simulink library "mcm_sil_M17_52_00_03_std"  (Simulink 8.3)
settings: Solver=ode45  StartTime=0.0  StopTime=10.0  RelTol=1e-3
undefined symbols (not defined in the file): sMP
libraries: MCM21_MDEG_EURO_10ms_wrapper x1
settings Model: Creator=PBASAVA  LastModifiedBy=PBASAVA

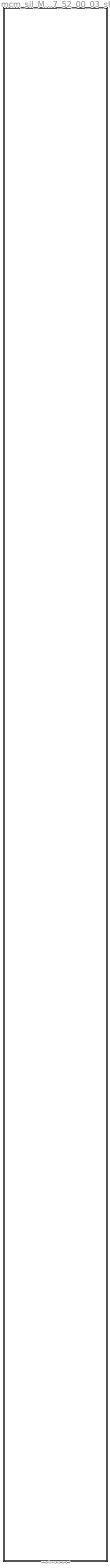
== system mcm_sil_M17_52_00_03_std ==
  mcm_sil_M17_52_00_03_std : Subsystem  mask{user_config=sMP.ctrl.mcm.user_config}

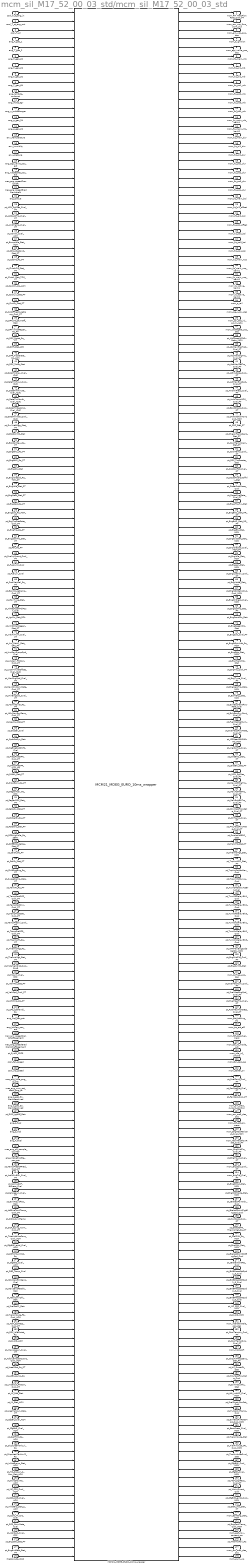
== system mcm_sil_M17_52_00_03_std/mcm_sil_M17_52_00_03_std ==
  cool_T_ct_eng_in : Inport
  cool_T_ct_eng_out : Inport  Port=2
  cool_T_oil : Inport  Port=3
  eng_T_gas_1 : Inport  Port=4
  eng_T_gas_2 : Inport  Port=5
  eng_T_gas_2N : Inport  Port=6
  eng_T_gas_2S : Inport  Port=7
  eng_T_gas_32 : Inport  Port=8
  eng_T_gas_6N : Inport  Port=9
  eng_lambda_exhaust : Inport  Port=10
  eng_mdot_egr : Inport  Port=11
  eng_n_turbocharger : Inport  Port=12
  eng_p_gas_2N : Inport  Port=13
  eng_p_gas_2S : Inport  Port=14
  env_Temperature : Inport  Port=15
  env_humidity : Inport  Port=16
  env_pressure : Inport  Port=17
  eng_egr_valve_pos_act : Inport  Port=18
  eng_wastegate_pos_act : Inport  Port=19
  mec_eng_speedCrankshaft : Inport  Port=20
  mec_eng_speedGradCrankshaft : Inport  Port=21
  eng_torque : Inport  Port=22
  pt_ACM_SglRes_Cval_PT : Inport  Port=23
  pt_ARRAddTrq_Cval_PT : Inport  Port=24
  pt_AmbTemp_Cval_PT : Inport  Port=25
  pt_AshVol_Cval_ACM : Inport  Port=26
  pt_BumpIdle_Stat_ACM : Inport  Port=27
  pt_CPC_IdleCond_Stat_PT : Inport  Port=28
  pt_CabHt_Rq_PT : Inport  Port=29
  pt_ClutchCls_Stat_PT : Inport  Port=30
  pt_Clutch_Stat_TCM_PT : Inport  Port=31
  pt_CoolDn_Rq_ACM : Inport  Port=32
  pt_CoolLvl_Stat_PT : Inport  Port=33
  pt_CurrGr_Stat_PT : Inport  Port=34
  pt_CutoffFreqSurgDamp_Cval_PT : Inport  Port=35
  pt_DPF_HC_BurnOff_Stat : Inport  Port=36
  pt_DPF_InhbtRegen_Rq_PT : Inport  Port=37
  pt_DPF_Protct_Rq_PT : Inport  Port=38
  pt_DPF_Stat_ACM : Inport  Port=39
  pt_DPF_TrqDerate_Rq_ACM : Inport  Port=40
  pt_DPF_Zone_Stat : Inport  Port=41
  pt_DateTmDay_Cval_ICUC : Inport  Port=42
  pt_DateTmHour_Cval_ICUC : Inport  Port=43
  pt_DateTmMinute_Cval_ICUC : Inport  Port=44
  pt_DateTmMonth_Cval_ICUC : Inport  Port=45
  pt_DateTmSecond_Cval_ICUC : Inport  Port=46
  pt_DateTmYear_Cval_ICUC : Inport  Port=47
  pt_DrvlineEngg_Stat_PT : Inport  Port=48
  pt_EcoRollMd_Stat : Inport  Port=49
  pt_EcoRollNeu_Rq_PT : Inport  Port=50
  pt_EngBrk1_Rq_PT : Inport  Port=51
  pt_EngBrk2_Rq_PT : Inport  Port=52
  pt_EngCrk_Stat : Inport  Port=53
  pt_EngIdleSpd_Rq_TCM_PT : Inport  Port=54
  pt_EngIdle_Stat_PT : Inport  Port=55
  pt_EngReSt_Stat_PT : Inport  Port=56
  pt_EngSpd_Rq_PT : Inport  Port=57
  pt_EngSpd_Rq_TCM_PT : Inport  Port=58
  pt_EngTrqDecRate_Cval_PT : Inport  Port=59
  pt_EngTrq_Rq_PT : Inport  Port=60
  pt_EngZeroTrq_Stat_PT : Inport  Port=61
  pt_Fan_Rq_PT : Inport  Port=62
  pt_FuelInjQuant_Cval_PT : Inport  Port=63
  pt_FuelLvl2_Cval : Inport  Port=64
  pt_FuelLvl_Cval : Inport  Port=65
  pt_FuelMapSel_Rq_PT : Inport  Port=66
  pt_GaimSurgDamp_Cval_PT : Inport  Port=67
  pt_GovType_Stat_PT : Inport  Port=68
  pt_HiResAccelPdlPosn_Cval : Inport  Port=69
  pt_IgnSw_Stat_SCA : Inport  Port=70
  pt_InhbtManRegen_Stat_PT : Inport  Port=71
  pt_IntkAirHum_Cval_PT : Inport  Port=72
  pt_Km_Parity_Stat_CPC_PT : Inport  Port=73
  pt_LimGovDroopSpd_Cval : Inport  Port=74
  pt_LmdaIn_FltrCorr_Cval_PT : Inport  Port=75
  pt_LocalMinuteOffset_Cval_ICUC : Inport  Port=76
  pt_MaxEngSpd_Cval_PT : Inport  Port=77
  pt_MaxNOxConvRate_Cval_PT : Inport  Port=78
  pt_MinEngSpd_Cval_PT : Inport  Port=79
  pt_MomntOver_Rq_PT : Inport  Port=80
  pt_NOxRawEmiSens_Cval_PT : Inport  Port=81
  pt_NeuSw_Stat_PT : Inport  Port=82
  pt_ObsSel_Cval : Inport  Port=83
  pt_OptIdleSys_Stat : Inport  Port=84
  pt_PreEngSpdShift_Cval : Inport  Port=85
  pt_PressPostDPF_Cval_PT : Inport  Port=86
  pt_PressPreDPF_Cval_PT : Inport  Port=87
  pt_PrkBrk_Stat_PT : Inport  Port=88
  pt_PropGain_Rq_PT : Inport  Port=89
  pt_RegenActv_Rq_CPC : Inport  Port=90
  pt_RegenDPF_Stat_PT : Inport  Port=91
  pt_RetActv_Stat_PT : Inport  Port=92
  pt_RlsSelGr_Rq_PT : Inport  Port=93
  pt_RotSens_Stat_PT : Inport  Port=94
  pt_SCRHighIdle_Rq_SERV : Inport  Port=95
  pt_SPEEDO_ZeSig_Stat_PT : Inport  Port=96
  pt_SelGr_Rq_PT : Inport  Port=97
  pt_SelGr_Stat_PT : Inport  Port=98
  pt_ShiftSprtEng_Rq_PT : Inport  Port=99
  pt_SurgeDamp_Stat_PT : Inport  Port=100
  pt_TankHt_Rq_PT : Inport  Port=101
  pt_TempPostDPF_Cval_PT : Inport  Port=102
  pt_TempPostOxi_Cval_PT : Inport  Port=103
  pt_TempPostSCR_Cval_PT : Inport  Port=104
  pt_TempPreOxi_Cval_PT : Inport  Port=105
  pt_TempPreSCR_Cval_PT : Inport  Port=106
  pt_ThermoHt_Rq_PT : Inport  Port=107
  pt_ThermoMgt_Rq_ACM : Inport  Port=108
  pt_ThermoMgt_Stat_PT : Inport  Port=109
  pt_TotalVehDist_Cval_DIAG : Inport  Port=110
  pt_TrqLim_Cval_CPC : Inport  Port=111
  pt_VehMtn_Stat_PT : Inport  Port=112
  pt_VehSpd_Cval_PT : Inport  Port=113
  pt_WtrPmp_Rq_PT : Inport  Port=114
  pt_ZPC_CstHandl_Rq : Inport  Port=115
  eng_vcp_pos_act : Inport  Port=116
  eng_brkflap_pos_act : Inport  Port=117
  mec_eng_speedCrankshaftSegment : Inport  Port=118
  mec_eng_speedGradCrankshaftSegment : Inport  Port=119
  pt_SysID_CPC3 : Inport  Port=120
  cool_fan_speed : Inport  Port=121
  cool_wp_speed : Inport  Port=122
  mec_eng_time_ang_cs_act : Inport  Port=123
  mec_eng_num_act_tooth_ang_cs : Inport  Port=124
  eng_p_gas_31_CrankResolved : Inport  Port=125
  eng_p_gas_32_CrankResolved : Inport  Port=126
  pt_DOC_LgtOff_Stat : Inport  Port=127
  eng_p_fuel : Inport  Port=128
  eng_p_hcd : Inport  Port=129
  eng_T_Fuel : Inport  Port=130
  mec_eng_p3_sample_counter : Inport  Port=131
  eng_intakethrottle_pos_act : Inport  Port=132
  pt_TempPreSCRPred_Cval_PT : Inport  Port=133
  pt_ActlNOxEmi_Cval_PT : Inport  Port=134
  pt_Norm_DPF_BkPress_Cval : Inport  Port=135
  pt_RelUreaLvl_Cval_PT : Inport  Port=136
  pt_ExhHtSysFlap_Stat : Inport  Port=137
  pt_AdBlueTankTemp_Cval_PT : Inport  Port=138
  pt_DOC_SyncTemp : Inport  Port=139
  pt_SCR_aging_norm_Cval_PT : Inport  Port=140
  pt_TotalAdblueCons_Cval_ACM : Inport  Port=141
  pt_CfgBit2_extd_Cval_ACM : Inport  Port=142
  pt_DPF_HC_Inhbt_Rq : Inport  Port=143
  pt_CfgBit2_Cval_ACM : Inport  Port=144
  pt_DEF_Temp_Cval : Inport  Port=145
  pt_NOxRawEmiSens_Cval : Inport  Port=146
  pt_NOxSensRatChk_Stat : Inport  Port=147
  pt_NOxConvChk_Stat : Inport  Port=148
  pt_FuelRefill_Stat : Inport  Port=149
  pt_Tier4Induce_FR_Cval_ACM : Inport  Port=150
  pt_ACM_SglRes2_Cval_PT : Inport  Port=151
  pt_DPF_IdleProtct_Rq : Inport  Port=152
  pt_SysID_ACM : Inport  Port=153
  pt_MaxUreaLvl_Cval_PT : Inport  Port=154
  pt_AdblueDoserQuant_Cval_ACM : Inport  Port=155
  pt_UreaDfrst_Rq_PT : Inport  Port=156
  pt_AdBlueLmp_Rq : Inport  Port=157
  pt_LmdaOut_FltrCorr_Cval_PT : Inport  Port=158
  pt_MI_Rds_Stat : Inport  Port=159
  pt_MI_Stat_ACM : Inport  Port=160
  pt_UreaTankLvl_Stat_PT : Inport  Port=161
  pt_CfgBit_Cval_ACM : Inport  Port=162
  pt_CfgBit3_Cval_ACM : Inport  Port=163
  pt_DelFMM_Rq_ACM : Inport  Port=164
  pt_DispUreaTankLvl_Rq : Inport  Port=165
  pt_DispUreaTankLvl2_Rq : Inport  Port=166
  pt_InhbtGroup_Stat_ACM : Inport  Port=167
  pt_HC_DosLvl_2_Mon_Stat_ACM : Inport  Port=168
  pt_FuncSftyVer_ACM : Inport  Port=169
  pt_MC_C29_Cval_ACM : Inport  Port=170
  pt_CRC_C29_Cval_ACM : Inport  Port=171
  pt_InhbtGrp_Stat_2_ACM : Inport  Port=172
  pt_Cont_MI_Cnt_Cval : Inport  Port=173
  pt_SCR_ConvRate_Cval : Inport  Port=174
  pt_VehSpd_Cval_CPC : Inport  Port=175
  pt_EngStrtr_Stat_PT : Inport  Port=176
  pt_EngExtStart_Stat_PT : Inport  Port=177
  PressAir_Rq_ICUC : Inport  Port=178
  MCM21_MDEG_EURO_10ms_wrapper : MCM21_MDEG_EURO_10ms_wrapper/MCM21_MDEG_EURO_10ms_wrapper  SystemSampleTime=-1
  mcm_PM_MassFlowRate_Cval_PT : Outport
  mcm_am_vcp_5ms_pwm_out : Outport  Port=2
  mcm_am_vcp_pos_des : Outport  Port=3
  mcm_b_ignition : Outport  Port=4
  mcm_egr_valve_pos_des : Outport  Port=5
  mcm_fis_main_mb : Outport  Port=6
  mcm_fis_pi1_mb : Outport  Port=7
  mcm_fis_pi2_mb : Outport  Port=8
  mcm_fis_po1_mb : Outport  Port=9
  mcm_fis_po2_mb : Outport  Port=10
  mcm_fis_po3_mb : Outport  Port=11
  mcm_fis_po4_mb : Outport  Port=12
  mcm_fis_main_mb_bank1 : Outport  Port=13
  mcm_fis_main_mb_bank2 : Outport  Port=14
  mcm_fis_main_dur : Outport  Port=15
  mcm_fis_pi1_dur : Outport  Port=16
  mcm_fis_pi2_dur : Outport  Port=17
  mcm_fis_po1_dur : Outport  Port=18
  mcm_fis_po2_dur : Outport  Port=19
  mcm_fis_po3_dur : Outport  Port=20
  mcm_fis_po4_dur : Outport  Port=21
  mcm_fis_main_boi : Outport  Port=22
  mcm_fis_pi1_offset : Outport  Port=23
  mcm_fis_pi2_boi : Outport  Port=24
  mcm_fis_po1_offset : Outport  Port=25
  mcm_fis_po2_boi : Outport  Port=26
  mcm_fis_po3_boi : Outport  Port=27
  mcm_fis_po4_boi : Outport  Port=28
  mcm_fis_main_nop : Outport  Port=29
  mcm_fis_main_nop_bank1 : Outport  Port=30
  mcm_fis_main_nop_bank2 : Outport  Port=31
  mcm_jb_active_bank1 : Outport  Port=32
  mcm_jb_active_bank2 : Outport  Port=33
  mcm_p_rail : Outport  Port=34
  mcm_rpg_i_pcv_des : Outport  Port=35
  mcm_spi_des_inj_asym_ratio : Outport  Port=36
  mcm_wastegate_pos_des : Outport  Port=37
  pt_ANCReadWFNOxRatio_MCM : Outport  Port=38
  pt_AbsMaxEngTrq2_Cval_PT : Outport  Port=39
  pt_AbsMaxEngTrq_Cval_PT : Outport  Port=40
  pt_AbsMaxRetTrq_Cval_PT : Outport  Port=41
  pt_ActlInjRate_Cval_PT : Outport  Port=42
  pt_ActlMaxEngSpd_Cval_PT : Outport  Port=43
  pt_AmbAirPress_Cval_PT : Outport  Port=44
  pt_AmbTempMCM_Cval_PT : Outport  Port=45
  pt_BoostPress_Cval_PT : Outport  Port=46
  pt_CANWrtGlblMonCond_MCM : Outport  Port=47
  pt_CPC_Stat_PT : Outport  Port=48
  pt_ChrgAirTempSens_Stat_PT : Outport  Port=49
  pt_CoolTempWarn_Stat_PT : Outport  Port=50
  pt_CoolTemp_Cval_PT : Outport  Port=51
  pt_DPF_TrqDerate_Stat : Outport  Port=52
  pt_DosCorrFctr_Cval_PT : Outport  Port=53
  pt_DoserFuelCutoffVlv_Stat : Outport  Port=54
  pt_DoserFuelPress_Cval : Outport  Port=55
  pt_DoserFuelRate_Cval_PT : Outport  Port=56
  pt_EngATS_Hw_Stat : Outport  Port=57
  pt_EngBrk1_Stat_MR_PT : Outport  Port=58
  pt_EngBrk2_Stat_MR_PT : Outport  Port=59
  pt_EngBrk_Stat_MCM : Outport  Port=60
  pt_EngExtStart_Stat_MCM : Outport  Port=61
  pt_EngIdleSpd_Cval_MCM_PT : Outport  Port=62
  pt_EngIdle_Stat_MCM : Outport  Port=63
  pt_EngIgn_Stat_MCM : Outport  Port=64
  pt_EngLoadIdx_Cval_PT : Outport  Port=65
  pt_EngMode_Stat_MCM : Outport  Port=66
  pt_EngNO2RatioOut_Cval_MCM : Outport  Port=67
  pt_EngOilPress_Cval_MCM : Outport  Port=68
  pt_EngOpPnt_Stat_PT : Outport  Port=69
  pt_EngPendRls_Stat : Outport  Port=70
  pt_EngRegenRls_Stat : Outport  Port=71
  pt_EngSpd_Cval_PT : Outport  Port=72
  pt_EngStSpInhbt_Rq_MCM : Outport  Port=73
  pt_EngStrtr_Stat_MCM : Outport  Port=74
  pt_EngTransMd_Stat : Outport  Port=75
  pt_EngTrq_Cval_PT : Outport  Port=76
  pt_EngType_Cval_PT : Outport  Port=77
  pt_EngZeroTrq_Stat_MCM : Outport  Port=78
  pt_EomEng_Stat_MCM : Outport  Port=79
  pt_ExhGasMassFlowRate_Cval : Outport  Port=80
  pt_ExhGasOxyCont_Cval_PT : Outport  Port=81
  pt_FuelMapSelNum_Cval_PT : Outport  Port=82
  pt_FuelMassFlowRate_Cval_PT : Outport  Port=83
  pt_ISPRead30GNOxMd_MCM : Outport  Port=84
  pt_InertiaTrq_Cval_PT : Outport  Port=85
  pt_JakeBrk2_Stat_PT : Outport  Port=86
  pt_JakeBrk_Stat_PT : Outport  Port=87
  pt_MCM_SglRes_Cval_PT : Outport  Port=88
  pt_MaxActlEngTrq_Cval_PT : Outport  Port=89
  pt_MaxActlRetTrq_Cval_PT : Outport  Port=90
  pt_MaxEngBrkTrq_Cval_PT : Outport  Port=91
  pt_NOxMassFlowRate_Cval_PT : Outport  Port=92
  pt_OilTemp_Cval_PT : Outport  Port=93
  pt_PM_MassFlowRate_Cval_PT : Outport  Port=94
  pt_SmokeMdEOP_Stat : Outport  Port=95
  pt_TankHt_Stat_PT : Outport  Port=96
  pt_ThermoMgt_Stat_MCM : Outport  Port=97
  pt_TrqLimNOx_Stat_PT : Outport  Port=98
  pt_TrqLimPctAbsMax_Cval : Outport  Port=99
  pt_TrqLimPctCurve_Cval : Outport  Port=100
  pt_TurnOffDelayActBrk_Cval : Outport  Port=101
  pt_TurnOffDelayBrk1_Cval : Outport  Port=102
  pt_TurnOffDelayBrk2_Cval : Outport  Port=103
  pt_TurnOffDelayBrk3_Cval : Outport  Port=104
  pt_TurnOnDelayBrk1_Cval : Outport  Port=105
  pt_TurnOnDelayBrk2_Cval : Outport  Port=106
  pt_TurnOnDelayBrk3_Cval : Outport  Port=107
  pt_WFAMaxEngSpd30gNOx_MCM : Outport  Port=108
  pt_EngFrictTrq_Cval_PT : Outport  Port=109
  pt_EngCylMd_Stat : Outport  Port=110
  mcm_brkflap_pos_des : Outport  Port=111
  pt_FuelMapNum_Cval_PT : Outport  Port=112
  pt_FuelMapEngSpd_Cval_PT : Outport  Port=113
  pt_FuelMapTrq_Cval_PT : Outport  Port=114
  pt_FuelMapTrqNoBst_Cval_PT : Outport  Port=115
  mcm_act_braking_trq : Outport  Port=116
  mcm_trq_act_eff : Outport  Port=117
  mcm_fbf_des_fuel_mass : Outport  Port=118
  mcm_tsa_itc_mode_act : Outport  Port=119
  mcm_wfa_wf_smoke : Outport  Port=120
  mcm_fan_spd_req : Outport  Port=121
  mcm_starter_on : Outport  Port=122
  pt_FuelCons_Cval_PT : Outport  Port=123
  pt_FanSpdPct_Cval_PT : Outport  Port=124
  pt_FanSpd_Cval_PT : Outport  Port=125
  mcm_am_sra3_current_position : Outport  Port=126
  mcm_am_sra3_des_pos : Outport  Port=127
  mcm_ccf_act_air_mass : Outport  Port=128
  mcm_EngNO2RatioOut_Cval_MCM : Outport  Port=129
  mcm_NOxMassFlowRate_Cval_PT : Outport  Port=130
  mcm_EngFrictTrq_Cval_PT : Outport  Port=131
  pt_EngHours_Cval_PT : Outport  Port=132
  mcm_EngSpd_Cval_PT : Outport  Port=133
  mcm_EngTrq_Cval_PT : Outport  Port=134
  pt_EngStrtrLk_Stat_MCM : Outport  Port=135
  pt_EngStrtrMode_Stat_MCM : Outport  Port=136
  pt_JBrakeSPointIdx_Cval : Outport  Port=137
  pt_JBrakeSPointTrgtEngSpd_Cval : Outport  Port=138
  pt_PwrClass_Cval_PT : Outport  Port=139
  pt_DeactDPF_ThermoMgt_Rq_PT : Outport  Port=140
  pt_DelFMM_Rq_MCM : Outport  Port=141
  pt_EngSNA_Stat_MCM : Outport  Port=142
  pt_JBrakeSPointStrtEngSpd_Cval : Outport  Port=143
  pt_JBrakeWghtFac_Cval : Outport  Port=144
  pt_JBrkBPressStrtSpd1_3_Cval : Outport  Port=145
  pt_JBrkBPressStrtSpd1_6_Cval : Outport  Port=146
  pt_JBrkBPressStrtSpd2_3_Cval : Outport  Port=147
  pt_JBrkBPressStrtSpd2_6_Cval : Outport  Port=148
  pt_MC_C02_Cval_MCM : Outport  Port=149
  pt_SysID_MCM : Outport  Port=150
  mcm_intakethrottle_pos_des : Outport  Port=151
  pt_CoolTempIn_Cval_PT : Outport  Port=152
  pt_CoolTempOut_Cval_PT : Outport  Port=153
  mcm_mdot_SFI : Outport  Port=154
  pt_ChrgAirPressSens_Stat_PT : Outport  Port=155
  pt_HC_DoserFlt_Stat : Outport  Port=156
  pt_PM_MassFlowRate_Cval : Outport  Port=157
  pt_ExhHtSysRls_Stat : Outport  Port=158
  pt_At1_IntkO2_Cval_MCM : Outport  Port=159
  pt_FuelDnstyCorrFctr_Cval : Outport  Port=160
  pt_TurboOutTemp_Cval : Outport  Port=161
  pt_ExhGasFlwRateMod_Cval_MCM : Outport  Port=162
  pt_BaroPress_Cval_MCM : Outport  Port=163
  pt_Tier4Induce_Stat : Outport  Port=164
  pt_Tier4Induce_FR_Cval_MCM : Outport  Port=165
  pt_Tier4InduceOvrd_Stat : Outport  Port=166
  pt_CfgBit2_Cval_MCM : Outport  Port=167
  pt_CfgBit_Cval_MCM : Outport  Port=168
  pt_MCM_SglRes2_Cval_PT : Outport  Port=169
  pt_WtrInjQuant_Cval : Outport  Port=170
  pt_CfgBit2_extd_Cval_MCM : Outport  Port=171
  pt_DEF_Lmp_Stat_PT : Outport  Port=172
  mcm_EomEng_Stat_MCM : Outport  Port=173
  pt_EngCoolTemp_Cval_MCM : Outport  Port=174
  mcm_eaf_nox_content_cor : Outport  Port=175
  pt_ThermoRoll_Rq : Outport  Port=176
  mcm_am_sra4_des_pos : Outport  Port=177
  mcm_pwm_wp : Outport  Port=178
  wires:
  cool_T_ct_eng_in/1 -> MCM21_MDEG_EURO_10ms_wrapper/1  "cool_T_ct_eng_in"
  cool_T_ct_eng_out/1 -> MCM21_MDEG_EURO_10ms_wrapper/2  "cool_T_ct_eng_out"
  cool_T_oil/1 -> MCM21_MDEG_EURO_10ms_wrapper/3  "cool_T_oil"
  eng_T_gas_1/1 -> MCM21_MDEG_EURO_10ms_wrapper/4  "eng_T_gas_1"
  eng_T_gas_2/1 -> MCM21_MDEG_EURO_10ms_wrapper/5  "eng_T_gas_2"
  eng_T_gas_2N/1 -> MCM21_MDEG_EURO_10ms_wrapper/6  "eng_T_gas_2N"
  eng_T_gas_2S/1 -> MCM21_MDEG_EURO_10ms_wrapper/7  "eng_T_gas_2S"
  eng_T_gas_32/1 -> MCM21_MDEG_EURO_10ms_wrapper/8  "eng_T_gas_32"
  eng_T_gas_6N/1 -> MCM21_MDEG_EURO_10ms_wrapper/9  "eng_T_gas_6N"
  eng_lambda_exhaust/1 -> MCM21_MDEG_EURO_10ms_wrapper/10  "eng_lambda_exhaust"
  eng_mdot_egr/1 -> MCM21_MDEG_EURO_10ms_wrapper/11  "eng_mdot_egr"
  eng_n_turbocharger/1 -> MCM21_MDEG_EURO_10ms_wrapper/12  "eng_n_turbocharger"
  eng_p_gas_2N/1 -> MCM21_MDEG_EURO_10ms_wrapper/13  "eng_p_gas_2N"
  eng_p_gas_2S/1 -> MCM21_MDEG_EURO_10ms_wrapper/14  "eng_p_gas_2S"
  env_Temperature/1 -> MCM21_MDEG_EURO_10ms_wrapper/15  "env_Temperature"
  env_humidity/1 -> MCM21_MDEG_EURO_10ms_wrapper/16  "env_humidity"
  env_pressure/1 -> MCM21_MDEG_EURO_10ms_wrapper/17  "env_pressure"
  eng_egr_valve_pos_act/1 -> MCM21_MDEG_EURO_10ms_wrapper/18  "eng_egr_valve_pos_act"
  eng_wastegate_pos_act/1 -> MCM21_MDEG_EURO_10ms_wrapper/19  "eng_wastegate_pos_act"
  mec_eng_speedCrankshaft/1 -> MCM21_MDEG_EURO_10ms_wrapper/20  "mec_eng_speedCrankshaft"
  mec_eng_speedGradCrankshaft/1 -> MCM21_MDEG_EURO_10ms_wrapper/21  "mec_eng_speedGradCrankshaft"
  eng_torque/1 -> MCM21_MDEG_EURO_10ms_wrapper/22  "eng_torque"
  pt_ACM_SglRes_Cval_PT/1 -> MCM21_MDEG_EURO_10ms_wrapper/23  "pt_ACM_SglRes_Cval_PT"
  pt_ARRAddTrq_Cval_PT/1 -> MCM21_MDEG_EURO_10ms_wrapper/24  "pt_ARRAddTrq_Cval_PT"
  pt_AmbTemp_Cval_PT/1 -> MCM21_MDEG_EURO_10ms_wrapper/25  "pt_AmbTemp_Cval_PT"
  pt_AshVol_Cval_ACM/1 -> MCM21_MDEG_EURO_10ms_wrapper/26  "pt_AshVol_Cval_ACM"
  pt_BumpIdle_Stat_ACM/1 -> MCM21_MDEG_EURO_10ms_wrapper/27  "pt_BumpIdle_Stat_ACM"
  pt_CPC_IdleCond_Stat_PT/1 -> MCM21_MDEG_EURO_10ms_wrapper/28  "pt_CPC_IdleCond_Stat_PT"
  pt_CabHt_Rq_PT/1 -> MCM21_MDEG_EURO_10ms_wrapper/29  "pt_CabHt_Rq_PT"
  pt_ClutchCls_Stat_PT/1 -> MCM21_MDEG_EURO_10ms_wrapper/30  "pt_ClutchCls_Stat_PT"
  pt_Clutch_Stat_TCM_PT/1 -> MCM21_MDEG_EURO_10ms_wrapper/31  "pt_Clutch_Stat_TCM_PT"
  pt_CoolDn_Rq_ACM/1 -> MCM21_MDEG_EURO_10ms_wrapper/32  "pt_CoolDn_Rq_ACM"
  pt_CoolLvl_Stat_PT/1 -> MCM21_MDEG_EURO_10ms_wrapper/33  "pt_CoolLvl_Stat_PT"
  pt_CurrGr_Stat_PT/1 -> MCM21_MDEG_EURO_10ms_wrapper/34  "pt_CurrGr_Stat_PT"
  pt_CutoffFreqSurgDamp_Cval_PT/1 -> MCM21_MDEG_EURO_10ms_wrapper/35  "pt_CutoffFreqSurgDamp_Cval_PT"
  pt_DPF_HC_BurnOff_Stat/1 -> MCM21_MDEG_EURO_10ms_wrapper/36  "pt_DPF_HC_BurnOff_Stat"
  pt_DPF_InhbtRegen_Rq_PT/1 -> MCM21_MDEG_EURO_10ms_wrapper/37  "pt_DPF_InhbtRegen_Rq_PT"
  pt_DPF_Protct_Rq_PT/1 -> MCM21_MDEG_EURO_10ms_wrapper/38  "pt_DPF_Protct_Rq_PT"
  pt_DPF_Stat_ACM/1 -> MCM21_MDEG_EURO_10ms_wrapper/39  "pt_DPF_Stat_ACM"
  pt_DPF_TrqDerate_Rq_ACM/1 -> MCM21_MDEG_EURO_10ms_wrapper/40  "pt_DPF_TrqDerate_Rq_ACM"
  pt_DPF_Zone_Stat/1 -> MCM21_MDEG_EURO_10ms_wrapper/41  "pt_DPF_Zone_Stat"
  pt_DateTmDay_Cval_ICUC/1 -> MCM21_MDEG_EURO_10ms_wrapper/42  "pt_DateTmDay_Cval_ICUC"
  pt_DateTmHour_Cval_ICUC/1 -> MCM21_MDEG_EURO_10ms_wrapper/43  "pt_DateTmHour_Cval_ICUC"
  pt_DateTmMinute_Cval_ICUC/1 -> MCM21_MDEG_EURO_10ms_wrapper/44  "pt_DateTmMinute_Cval_ICUC"
  pt_DateTmMonth_Cval_ICUC/1 -> MCM21_MDEG_EURO_10ms_wrapper/45  "pt_DateTmMonth_Cval_ICUC"
  pt_DateTmSecond_Cval_ICUC/1 -> MCM21_MDEG_EURO_10ms_wrapper/46  "pt_DateTmSecond_Cval_ICUC"
  pt_DateTmYear_Cval_ICUC/1 -> MCM21_MDEG_EURO_10ms_wrapper/47  "pt_DateTmYear_Cval_ICUC"
  pt_DrvlineEngg_Stat_PT/1 -> MCM21_MDEG_EURO_10ms_wrapper/48  "pt_DrvlineEngg_Stat_PT"
  pt_EcoRollMd_Stat/1 -> MCM21_MDEG_EURO_10ms_wrapper/49  "pt_EcoRollMd_Stat"
  pt_EcoRollNeu_Rq_PT/1 -> MCM21_MDEG_EURO_10ms_wrapper/50  "pt_EcoRollNeu_Rq_PT"
  pt_EngBrk1_Rq_PT/1 -> MCM21_MDEG_EURO_10ms_wrapper/51  "pt_EngBrk1_Rq_PT"
  pt_EngBrk2_Rq_PT/1 -> MCM21_MDEG_EURO_10ms_wrapper/52  "pt_EngBrk2_Rq_PT"
  pt_EngCrk_Stat/1 -> MCM21_MDEG_EURO_10ms_wrapper/53  "pt_EngCrk_Stat"
  pt_EngIdleSpd_Rq_TCM_PT/1 -> MCM21_MDEG_EURO_10ms_wrapper/54  "pt_EngIdleSpd_Rq_TCM_PT"
  pt_EngIdle_Stat_PT/1 -> MCM21_MDEG_EURO_10ms_wrapper/55  "pt_EngIdle_Stat_PT"
  pt_EngReSt_Stat_PT/1 -> MCM21_MDEG_EURO_10ms_wrapper/56  "pt_EngReSt_Stat_PT"
  pt_EngSpd_Rq_PT/1 -> MCM21_MDEG_EURO_10ms_wrapper/57  "pt_EngSpd_Rq_PT"
  pt_EngSpd_Rq_TCM_PT/1 -> MCM21_MDEG_EURO_10ms_wrapper/58  "pt_EngSpd_Rq_TCM_PT"
  pt_EngTrqDecRate_Cval_PT/1 -> MCM21_MDEG_EURO_10ms_wrapper/59  "pt_EngTrqDecRate_Cval_PT"
  pt_EngTrq_Rq_PT/1 -> MCM21_MDEG_EURO_10ms_wrapper/60  "pt_EngTrq_Rq_PT"
  pt_EngZeroTrq_Stat_PT/1 -> MCM21_MDEG_EURO_10ms_wrapper/61  "pt_EngZeroTrq_Stat_PT"
  pt_Fan_Rq_PT/1 -> MCM21_MDEG_EURO_10ms_wrapper/62  "pt_Fan_Rq_PT"
  pt_FuelInjQuant_Cval_PT/1 -> MCM21_MDEG_EURO_10ms_wrapper/63  "pt_FuelInjQuant_Cval_PT"
  pt_FuelLvl2_Cval/1 -> MCM21_MDEG_EURO_10ms_wrapper/64  "pt_FuelLvl2_Cval"
  pt_FuelLvl_Cval/1 -> MCM21_MDEG_EURO_10ms_wrapper/65  "pt_FuelLvl_Cval"
  pt_FuelMapSel_Rq_PT/1 -> MCM21_MDEG_EURO_10ms_wrapper/66  "pt_FuelMapSel_Rq_PT"
  pt_GaimSurgDamp_Cval_PT/1 -> MCM21_MDEG_EURO_10ms_wrapper/67  "pt_GaimSurgDamp_Cval_PT"
  pt_GovType_Stat_PT/1 -> MCM21_MDEG_EURO_10ms_wrapper/68  "pt_GovType_Stat_PT"
  pt_HiResAccelPdlPosn_Cval/1 -> MCM21_MDEG_EURO_10ms_wrapper/69  "pt_HiResAccelPdlPosn_Cval"
  pt_IgnSw_Stat_SCA/1 -> MCM21_MDEG_EURO_10ms_wrapper/70  "pt_IgnSw_Stat_SCA"
  pt_InhbtManRegen_Stat_PT/1 -> MCM21_MDEG_EURO_10ms_wrapper/71  "pt_InhbtManRegen_Stat_PT"
  pt_IntkAirHum_Cval_PT/1 -> MCM21_MDEG_EURO_10ms_wrapper/72  "pt_IntkAirHum_Cval_PT"
  pt_Km_Parity_Stat_CPC_PT/1 -> MCM21_MDEG_EURO_10ms_wrapper/73  "pt_Km_Parity_Stat_CPC_PT"
  pt_LimGovDroopSpd_Cval/1 -> MCM21_MDEG_EURO_10ms_wrapper/74  "pt_LimGovDroopSpd_Cval"
  pt_LmdaIn_FltrCorr_Cval_PT/1 -> MCM21_MDEG_EURO_10ms_wrapper/75  "pt_LmdaIn_FltrCorr_Cval_PT"
  pt_LocalMinuteOffset_Cval_ICUC/1 -> MCM21_MDEG_EURO_10ms_wrapper/76  "pt_LocalMinuteOffset_Cval_ICUC"
  pt_MaxEngSpd_Cval_PT/1 -> MCM21_MDEG_EURO_10ms_wrapper/77  "pt_MaxEngSpd_Cval_PT"
  pt_MaxNOxConvRate_Cval_PT/1 -> MCM21_MDEG_EURO_10ms_wrapper/78  "pt_MaxNOxConvRate_Cval_PT"
  pt_MinEngSpd_Cval_PT/1 -> MCM21_MDEG_EURO_10ms_wrapper/79  "pt_MinEngSpd_Cval_PT"
  pt_MomntOver_Rq_PT/1 -> MCM21_MDEG_EURO_10ms_wrapper/80  "pt_MomntOver_Rq_PT"
  pt_NOxRawEmiSens_Cval_PT/1 -> MCM21_MDEG_EURO_10ms_wrapper/81  "pt_NOxRawEmiSens_Cval_PT"
  pt_NeuSw_Stat_PT/1 -> MCM21_MDEG_EURO_10ms_wrapper/82  "pt_NeuSw_Stat_PT"
  pt_ObsSel_Cval/1 -> MCM21_MDEG_EURO_10ms_wrapper/83  "pt_ObsSel_Cval"
  pt_OptIdleSys_Stat/1 -> MCM21_MDEG_EURO_10ms_wrapper/84  "pt_OptIdleSys_Stat"
  pt_PreEngSpdShift_Cval/1 -> MCM21_MDEG_EURO_10ms_wrapper/85  "pt_PreEngSpdShift_Cval"
  pt_PressPostDPF_Cval_PT/1 -> MCM21_MDEG_EURO_10ms_wrapper/86  "pt_PressPostDPF_Cval_PT"
  pt_PressPreDPF_Cval_PT/1 -> MCM21_MDEG_EURO_10ms_wrapper/87  "pt_PressPreDPF_Cval_PT"
  pt_PrkBrk_Stat_PT/1 -> MCM21_MDEG_EURO_10ms_wrapper/88  "pt_PrkBrk_Stat_PT"
  pt_PropGain_Rq_PT/1 -> MCM21_MDEG_EURO_10ms_wrapper/89  "pt_PropGain_Rq_PT"
  pt_RegenActv_Rq_CPC/1 -> MCM21_MDEG_EURO_10ms_wrapper/90  "pt_RegenActv_Rq_CPC"
  pt_RegenDPF_Stat_PT/1 -> MCM21_MDEG_EURO_10ms_wrapper/91  "pt_RegenDPF_Stat_PT"
  pt_RetActv_Stat_PT/1 -> MCM21_MDEG_EURO_10ms_wrapper/92  "pt_RetActv_Stat_PT"
  pt_RlsSelGr_Rq_PT/1 -> MCM21_MDEG_EURO_10ms_wrapper/93  "pt_RlsSelGr_Rq_PT"
  pt_RotSens_Stat_PT/1 -> MCM21_MDEG_EURO_10ms_wrapper/94  "pt_RotSens_Stat_PT"
  pt_SCRHighIdle_Rq_SERV/1 -> MCM21_MDEG_EURO_10ms_wrapper/95  "pt_SCRHighIdle_Rq_SERV"
  pt_SPEEDO_ZeSig_Stat_PT/1 -> MCM21_MDEG_EURO_10ms_wrapper/96  "pt_SPEEDO_ZeSig_Stat_PT"
  pt_SelGr_Rq_PT/1 -> MCM21_MDEG_EURO_10ms_wrapper/97  "pt_SelGr_Rq_PT"
  pt_SelGr_Stat_PT/1 -> MCM21_MDEG_EURO_10ms_wrapper/98  "pt_SelGr_Stat_PT"
  pt_ShiftSprtEng_Rq_PT/1 -> MCM21_MDEG_EURO_10ms_wrapper/99  "pt_ShiftSprtEng_Rq_PT"
  pt_SurgeDamp_Stat_PT/1 -> MCM21_MDEG_EURO_10ms_wrapper/100  "pt_SurgeDamp_Stat_PT"
  pt_TankHt_Rq_PT/1 -> MCM21_MDEG_EURO_10ms_wrapper/101  "pt_TankHt_Rq_PT"
  pt_TempPostDPF_Cval_PT/1 -> MCM21_MDEG_EURO_10ms_wrapper/102  "pt_TempPostDPF_Cval_PT"
  pt_TempPostOxi_Cval_PT/1 -> MCM21_MDEG_EURO_10ms_wrapper/103  "pt_TempPostOxi_Cval_PT"
  pt_TempPostSCR_Cval_PT/1 -> MCM21_MDEG_EURO_10ms_wrapper/104  "pt_TempPostSCR_Cval_PT"
  pt_TempPreOxi_Cval_PT/1 -> MCM21_MDEG_EURO_10ms_wrapper/105  "pt_TempPreOxi_Cval_PT"
  pt_TempPreSCR_Cval_PT/1 -> MCM21_MDEG_EURO_10ms_wrapper/106  "pt_TempPreSCR_Cval_PT"
  pt_ThermoHt_Rq_PT/1 -> MCM21_MDEG_EURO_10ms_wrapper/107  "pt_ThermoHt_Rq_PT"
  pt_ThermoMgt_Rq_ACM/1 -> MCM21_MDEG_EURO_10ms_wrapper/108  "pt_ThermoMgt_Rq_ACM"
  pt_ThermoMgt_Stat_PT/1 -> MCM21_MDEG_EURO_10ms_wrapper/109  "pt_ThermoMgt_Stat_PT"
  pt_TotalVehDist_Cval_DIAG/1 -> MCM21_MDEG_EURO_10ms_wrapper/110  "pt_TotalVehDist_Cval_DIAG"
  pt_TrqLim_Cval_CPC/1 -> MCM21_MDEG_EURO_10ms_wrapper/111  "pt_TrqLim_Cval_CPC"
  pt_VehMtn_Stat_PT/1 -> MCM21_MDEG_EURO_10ms_wrapper/112  "pt_VehMtn_Stat_PT"
  pt_VehSpd_Cval_PT/1 -> MCM21_MDEG_EURO_10ms_wrapper/113  "pt_VehSpd_Cval_PT"
  pt_WtrPmp_Rq_PT/1 -> MCM21_MDEG_EURO_10ms_wrapper/114  "pt_WtrPmp_Rq_PT"
  pt_ZPC_CstHandl_Rq/1 -> MCM21_MDEG_EURO_10ms_wrapper/115  "pt_ZPC_CstHandl_Rq"
  eng_vcp_pos_act/1 -> MCM21_MDEG_EURO_10ms_wrapper/116  "eng_vcp_pos_act"
  eng_brkflap_pos_act/1 -> MCM21_MDEG_EURO_10ms_wrapper/117  "eng_brkflap_pos_act"
  mec_eng_speedCrankshaftSegment/1 -> MCM21_MDEG_EURO_10ms_wrapper/118  "mec_eng_speedCrankshaftSegment"
  mec_eng_speedGradCrankshaftSegment/1 -> MCM21_MDEG_EURO_10ms_wrapper/119  "mec_eng_speedGradCrankshaftSegment"
  pt_SysID_CPC3/1 -> MCM21_MDEG_EURO_10ms_wrapper/120  "pt_SysID_CPC3"
  cool_fan_speed/1 -> MCM21_MDEG_EURO_10ms_wrapper/121  "cool_fan_speed"
  cool_wp_speed/1 -> MCM21_MDEG_EURO_10ms_wrapper/122  "cool_wp_speed"
  mec_eng_time_ang_cs_act/1 -> MCM21_MDEG_EURO_10ms_wrapper/123  "mec_eng_time_ang_cs_act"
  mec_eng_num_act_tooth_ang_cs/1 -> MCM21_MDEG_EURO_10ms_wrapper/124  "mec_eng_num_act_tooth_ang_cs"
  eng_p_gas_31_CrankResolved/1 -> MCM21_MDEG_EURO_10ms_wrapper/125  "eng_p_gas_31_CrankResolved"
  eng_p_gas_32_CrankResolved/1 -> MCM21_MDEG_EURO_10ms_wrapper/126  "eng_p_gas_32_CrankResolved"
  pt_DOC_LgtOff_Stat/1 -> MCM21_MDEG_EURO_10ms_wrapper/127  "pt_DOC_LgtOff_Stat"
  eng_p_fuel/1 -> MCM21_MDEG_EURO_10ms_wrapper/128  "eng_p_fuel"
  eng_p_hcd/1 -> MCM21_MDEG_EURO_10ms_wrapper/129  "eng_p_hcd"
  eng_T_Fuel/1 -> MCM21_MDEG_EURO_10ms_wrapper/130  "eng_T_Fuel"
  mec_eng_p3_sample_counter/1 -> MCM21_MDEG_EURO_10ms_wrapper/131  "mec_eng_p3_sample_counter"
  eng_intakethrottle_pos_act/1 -> MCM21_MDEG_EURO_10ms_wrapper/132  "eng_intakethrottle_pos_act"
  pt_TempPreSCRPred_Cval_PT/1 -> MCM21_MDEG_EURO_10ms_wrapper/133  "pt_TempPreSCRPred_Cval_PT"
  pt_ActlNOxEmi_Cval_PT/1 -> MCM21_MDEG_EURO_10ms_wrapper/134  "pt_ActlNOxEmi_Cval_PT"
  pt_Norm_DPF_BkPress_Cval/1 -> MCM21_MDEG_EURO_10ms_wrapper/135  "pt_Norm_DPF_BkPress_Cval"
  pt_RelUreaLvl_Cval_PT/1 -> MCM21_MDEG_EURO_10ms_wrapper/136  "pt_RelUreaLvl_Cval_PT"
  pt_ExhHtSysFlap_Stat/1 -> MCM21_MDEG_EURO_10ms_wrapper/137  "pt_ExhHtSysFlap_Stat"
  pt_AdBlueTankTemp_Cval_PT/1 -> MCM21_MDEG_EURO_10ms_wrapper/138  "pt_AdBlueTankTemp_Cval_PT"
  pt_DOC_SyncTemp/1 -> MCM21_MDEG_EURO_10ms_wrapper/139  "pt_DOC_SyncTemp"
  pt_SCR_aging_norm_Cval_PT/1 -> MCM21_MDEG_EURO_10ms_wrapper/140  "pt_SCR_aging_norm_Cval_PT"
  pt_TotalAdblueCons_Cval_ACM/1 -> MCM21_MDEG_EURO_10ms_wrapper/141  "pt_TotalAdblueCons_Cval_ACM"
  pt_CfgBit2_extd_Cval_ACM/1 -> MCM21_MDEG_EURO_10ms_wrapper/142  "pt_CfgBit2_extd_Cval_ACM"
  pt_DPF_HC_Inhbt_Rq/1 -> MCM21_MDEG_EURO_10ms_wrapper/143  "pt_DPF_HC_Inhbt_Rq"
  pt_CfgBit2_Cval_ACM/1 -> MCM21_MDEG_EURO_10ms_wrapper/144  "pt_CfgBit2_Cval_ACM"
  pt_DEF_Temp_Cval/1 -> MCM21_MDEG_EURO_10ms_wrapper/145  "pt_DEF_Temp_Cval"
  pt_NOxRawEmiSens_Cval/1 -> MCM21_MDEG_EURO_10ms_wrapper/146  "pt_NOxRawEmiSens_Cval"
  pt_NOxSensRatChk_Stat/1 -> MCM21_MDEG_EURO_10ms_wrapper/147  "pt_NOxSensRatChk_Stat"
  pt_NOxConvChk_Stat/1 -> MCM21_MDEG_EURO_10ms_wrapper/148  "pt_NOxConvChk_Stat"
  pt_FuelRefill_Stat/1 -> MCM21_MDEG_EURO_10ms_wrapper/149  "pt_FuelRefill_Stat"
  pt_Tier4Induce_FR_Cval_ACM/1 -> MCM21_MDEG_EURO_10ms_wrapper/150  "pt_Tier4Induce_FR_Cval_ACM"
  pt_ACM_SglRes2_Cval_PT/1 -> MCM21_MDEG_EURO_10ms_wrapper/151  "pt_ACM_SglRes2_Cval_PT"
  pt_DPF_IdleProtct_Rq/1 -> MCM21_MDEG_EURO_10ms_wrapper/152  "pt_DPF_IdleProtct_Rq"
  pt_SysID_ACM/1 -> MCM21_MDEG_EURO_10ms_wrapper/153  "pt_SysID_ACM"
  pt_MaxUreaLvl_Cval_PT/1 -> MCM21_MDEG_EURO_10ms_wrapper/154  "pt_MaxUreaLvl_Cval_PT"
  pt_AdblueDoserQuant_Cval_ACM/1 -> MCM21_MDEG_EURO_10ms_wrapper/155  "pt_AdblueDoserQuant_Cval_ACM"
  pt_UreaDfrst_Rq_PT/1 -> MCM21_MDEG_EURO_10ms_wrapper/156  "pt_UreaDfrst_Rq_PT"
  pt_AdBlueLmp_Rq/1 -> MCM21_MDEG_EURO_10ms_wrapper/157  "pt_AdBlueLmp_Rq"
  pt_LmdaOut_FltrCorr_Cval_PT/1 -> MCM21_MDEG_EURO_10ms_wrapper/158  "pt_LmdaOut_FltrCorr_Cval_PT"
  pt_MI_Rds_Stat/1 -> MCM21_MDEG_EURO_10ms_wrapper/159  "pt_MI_Rds_Stat"
  pt_MI_Stat_ACM/1 -> MCM21_MDEG_EURO_10ms_wrapper/160  "pt_MI_Stat_ACM"
  pt_UreaTankLvl_Stat_PT/1 -> MCM21_MDEG_EURO_10ms_wrapper/161  "pt_UreaTankLvl_Stat_PT"
  pt_CfgBit_Cval_ACM/1 -> MCM21_MDEG_EURO_10ms_wrapper/162  "pt_CfgBit_Cval_ACM"
  pt_CfgBit3_Cval_ACM/1 -> MCM21_MDEG_EURO_10ms_wrapper/163  "pt_CfgBit3_Cval_ACM"
  pt_DelFMM_Rq_ACM/1 -> MCM21_MDEG_EURO_10ms_wrapper/164  "pt_DelFMM_Rq_ACM"
  pt_DispUreaTankLvl_Rq/1 -> MCM21_MDEG_EURO_10ms_wrapper/165  "pt_DispUreaTankLvl_Rq"
  pt_DispUreaTankLvl2_Rq/1 -> MCM21_MDEG_EURO_10ms_wrapper/166  "pt_DispUreaTankLvl2_Rq"
  pt_InhbtGroup_Stat_ACM/1 -> MCM21_MDEG_EURO_10ms_wrapper/167  "pt_InhbtGroup_Stat_ACM"
  pt_HC_DosLvl_2_Mon_Stat_ACM/1 -> MCM21_MDEG_EURO_10ms_wrapper/168  "pt_HC_DosLvl_2_Mon_Stat_ACM"
  pt_FuncSftyVer_ACM/1 -> MCM21_MDEG_EURO_10ms_wrapper/169  "pt_FuncSftyVer_ACM"
  pt_MC_C29_Cval_ACM/1 -> MCM21_MDEG_EURO_10ms_wrapper/170  "pt_MC_C29_Cval_ACM"
  pt_CRC_C29_Cval_ACM/1 -> MCM21_MDEG_EURO_10ms_wrapper/171  "pt_CRC_C29_Cval_ACM"
  pt_InhbtGrp_Stat_2_ACM/1 -> MCM21_MDEG_EURO_10ms_wrapper/172  "pt_InhbtGrp_Stat_2_ACM"
  pt_Cont_MI_Cnt_Cval/1 -> MCM21_MDEG_EURO_10ms_wrapper/173  "pt_Cont_MI_Cnt_Cval"
  pt_SCR_ConvRate_Cval/1 -> MCM21_MDEG_EURO_10ms_wrapper/174  "pt_SCR_ConvRate_Cval"
  pt_VehSpd_Cval_CPC/1 -> MCM21_MDEG_EURO_10ms_wrapper/175  "pt_VehSpd_Cval_CPC"
  pt_EngStrtr_Stat_PT/1 -> MCM21_MDEG_EURO_10ms_wrapper/176  "pt_EngStrtr_Stat_PT"
  pt_EngExtStart_Stat_PT/1 -> MCM21_MDEG_EURO_10ms_wrapper/177  "pt_EngExtStart_Stat_PT"
  PressAir_Rq_ICUC/1 -> MCM21_MDEG_EURO_10ms_wrapper/178  "PressAir_Rq_ICUC"
  MCM21_MDEG_EURO_10ms_wrapper/1 -> mcm_PM_MassFlowRate_Cval_PT/1  "mcm_PM_MassFlowRate_Cval_PT"
  MCM21_MDEG_EURO_10ms_wrapper/2 -> mcm_am_vcp_5ms_pwm_out/1  "mcm_am_vcp_5ms_pwm_out"
  MCM21_MDEG_EURO_10ms_wrapper/3 -> mcm_am_vcp_pos_des/1  "mcm_am_vcp_pos_des"
  MCM21_MDEG_EURO_10ms_wrapper/4 -> mcm_b_ignition/1  "mcm_b_ignition"
  MCM21_MDEG_EURO_10ms_wrapper/5 -> mcm_egr_valve_pos_des/1  "mcm_egr_valve_pos_des"
  MCM21_MDEG_EURO_10ms_wrapper/6 -> mcm_fis_main_mb/1  "mcm_fis_main_mb"
  MCM21_MDEG_EURO_10ms_wrapper/7 -> mcm_fis_pi1_mb/1  "mcm_fis_pi1_mb"
  MCM21_MDEG_EURO_10ms_wrapper/8 -> mcm_fis_pi2_mb/1  "mcm_fis_pi2_mb"
  MCM21_MDEG_EURO_10ms_wrapper/9 -> mcm_fis_po1_mb/1  "mcm_fis_po1_mb"
  MCM21_MDEG_EURO_10ms_wrapper/10 -> mcm_fis_po2_mb/1  "mcm_fis_po2_mb"
  MCM21_MDEG_EURO_10ms_wrapper/11 -> mcm_fis_po3_mb/1  "mcm_fis_po3_mb"
  MCM21_MDEG_EURO_10ms_wrapper/12 -> mcm_fis_po4_mb/1  "mcm_fis_po4_mb"
  MCM21_MDEG_EURO_10ms_wrapper/13 -> mcm_fis_main_mb_bank1/1  "mcm_fis_main_mb_bank1"
  MCM21_MDEG_EURO_10ms_wrapper/14 -> mcm_fis_main_mb_bank2/1  "mcm_fis_main_mb_bank2"
  MCM21_MDEG_EURO_10ms_wrapper/15 -> mcm_fis_main_dur/1  "mcm_fis_main_dur"
  MCM21_MDEG_EURO_10ms_wrapper/16 -> mcm_fis_pi1_dur/1  "mcm_fis_pi1_dur"
  MCM21_MDEG_EURO_10ms_wrapper/17 -> mcm_fis_pi2_dur/1  "mcm_fis_pi2_dur"
  MCM21_MDEG_EURO_10ms_wrapper/18 -> mcm_fis_po1_dur/1  "mcm_fis_po1_dur"
  MCM21_MDEG_EURO_10ms_wrapper/19 -> mcm_fis_po2_dur/1  "mcm_fis_po2_dur"
  MCM21_MDEG_EURO_10ms_wrapper/20 -> mcm_fis_po3_dur/1  "mcm_fis_po3_dur"
  MCM21_MDEG_EURO_10ms_wrapper/21 -> mcm_fis_po4_dur/1  "mcm_fis_po4_dur"
  MCM21_MDEG_EURO_10ms_wrapper/22 -> mcm_fis_main_boi/1  "mcm_fis_main_boi"
  MCM21_MDEG_EURO_10ms_wrapper/23 -> mcm_fis_pi1_offset/1  "mcm_fis_pi1_offset"
  MCM21_MDEG_EURO_10ms_wrapper/24 -> mcm_fis_pi2_boi/1  "mcm_fis_pi2_boi"
  MCM21_MDEG_EURO_10ms_wrapper/25 -> mcm_fis_po1_offset/1  "mcm_fis_po1_offset"
  MCM21_MDEG_EURO_10ms_wrapper/26 -> mcm_fis_po2_boi/1  "mcm_fis_po2_boi"
  MCM21_MDEG_EURO_10ms_wrapper/27 -> mcm_fis_po3_boi/1  "mcm_fis_po3_boi"
  MCM21_MDEG_EURO_10ms_wrapper/28 -> mcm_fis_po4_boi/1  "mcm_fis_po4_boi"
  MCM21_MDEG_EURO_10ms_wrapper/29 -> mcm_fis_main_nop/1  "mcm_fis_main_nop"
  MCM21_MDEG_EURO_10ms_wrapper/30 -> mcm_fis_main_nop_bank1/1  "mcm_fis_main_nop_bank1"
  MCM21_MDEG_EURO_10ms_wrapper/31 -> mcm_fis_main_nop_bank2/1  "mcm_fis_main_nop_bank2"
  MCM21_MDEG_EURO_10ms_wrapper/32 -> mcm_jb_active_bank1/1  "mcm_jb_active_bank1"
  MCM21_MDEG_EURO_10ms_wrapper/33 -> mcm_jb_active_bank2/1  "mcm_jb_active_bank2"
  MCM21_MDEG_EURO_10ms_wrapper/34 -> mcm_p_rail/1  "mcm_p_rail"
  MCM21_MDEG_EURO_10ms_wrapper/35 -> mcm_rpg_i_pcv_des/1  "mcm_rpg_i_pcv_des"
  MCM21_MDEG_EURO_10ms_wrapper/36 -> mcm_spi_des_inj_asym_ratio/1  "mcm_spi_des_inj_asym_ratio"
  MCM21_MDEG_EURO_10ms_wrapper/37 -> mcm_wastegate_pos_des/1  "mcm_wastegate_pos_des"
  MCM21_MDEG_EURO_10ms_wrapper/38 -> pt_ANCReadWFNOxRatio_MCM/1  "pt_ANCReadWFNOxRatio_MCM"
  MCM21_MDEG_EURO_10ms_wrapper/39 -> pt_AbsMaxEngTrq2_Cval_PT/1  "pt_AbsMaxEngTrq2_Cval_PT"
  MCM21_MDEG_EURO_10ms_wrapper/40 -> pt_AbsMaxEngTrq_Cval_PT/1  "pt_AbsMaxEngTrq_Cval_PT"
  MCM21_MDEG_EURO_10ms_wrapper/41 -> pt_AbsMaxRetTrq_Cval_PT/1  "pt_AbsMaxRetTrq_Cval_PT"
  MCM21_MDEG_EURO_10ms_wrapper/42 -> pt_ActlInjRate_Cval_PT/1  "pt_ActlInjRate_Cval_PT"
  MCM21_MDEG_EURO_10ms_wrapper/43 -> pt_ActlMaxEngSpd_Cval_PT/1  "pt_ActlMaxEngSpd_Cval_PT"
  MCM21_MDEG_EURO_10ms_wrapper/44 -> pt_AmbAirPress_Cval_PT/1  "pt_AmbAirPress_Cval_PT"
  MCM21_MDEG_EURO_10ms_wrapper/45 -> pt_AmbTempMCM_Cval_PT/1  "pt_AmbTempMCM_Cval_PT"
  MCM21_MDEG_EURO_10ms_wrapper/46 -> pt_BoostPress_Cval_PT/1  "pt_BoostPress_Cval_PT"
  MCM21_MDEG_EURO_10ms_wrapper/47 -> pt_CANWrtGlblMonCond_MCM/1  "pt_CANWrtGlblMonCond_MCM"
  MCM21_MDEG_EURO_10ms_wrapper/48 -> pt_CPC_Stat_PT/1  "pt_CPC_Stat_PT"
  MCM21_MDEG_EURO_10ms_wrapper/49 -> pt_ChrgAirTempSens_Stat_PT/1  "pt_ChrgAirTempSens_Stat_PT"
  MCM21_MDEG_EURO_10ms_wrapper/50 -> pt_CoolTempWarn_Stat_PT/1  "pt_CoolTempWarn_Stat_PT"
  MCM21_MDEG_EURO_10ms_wrapper/51 -> pt_CoolTemp_Cval_PT/1  "pt_CoolTemp_Cval_PT"
  MCM21_MDEG_EURO_10ms_wrapper/52 -> pt_DPF_TrqDerate_Stat/1  "pt_DPF_TrqDerate_Stat"
  MCM21_MDEG_EURO_10ms_wrapper/53 -> pt_DosCorrFctr_Cval_PT/1  "pt_DosCorrFctr_Cval_PT"
  MCM21_MDEG_EURO_10ms_wrapper/54 -> pt_DoserFuelCutoffVlv_Stat/1  "pt_DoserFuelCutoffVlv_Stat"
  MCM21_MDEG_EURO_10ms_wrapper/55 -> pt_DoserFuelPress_Cval/1  "pt_DoserFuelPress_Cval"
  MCM21_MDEG_EURO_10ms_wrapper/56 -> pt_DoserFuelRate_Cval_PT/1  "pt_DoserFuelRate_Cval_PT"
  MCM21_MDEG_EURO_10ms_wrapper/57 -> pt_EngATS_Hw_Stat/1  "pt_EngATS_Hw_Stat"
  MCM21_MDEG_EURO_10ms_wrapper/58 -> pt_EngBrk1_Stat_MR_PT/1  "pt_EngBrk1_Stat_MR_PT"
  MCM21_MDEG_EURO_10ms_wrapper/59 -> pt_EngBrk2_Stat_MR_PT/1  "pt_EngBrk2_Stat_MR_PT"
  MCM21_MDEG_EURO_10ms_wrapper/60 -> pt_EngBrk_Stat_MCM/1  "pt_EngBrk_Stat_MCM"
  MCM21_MDEG_EURO_10ms_wrapper/61 -> pt_EngExtStart_Stat_MCM/1  "pt_EngExtStart_Stat_MCM"
  MCM21_MDEG_EURO_10ms_wrapper/62 -> pt_EngIdleSpd_Cval_MCM_PT/1  "pt_EngIdleSpd_Cval_MCM_PT"
  MCM21_MDEG_EURO_10ms_wrapper/63 -> pt_EngIdle_Stat_MCM/1  "pt_EngIdle_Stat_MCM"
  MCM21_MDEG_EURO_10ms_wrapper/64 -> pt_EngIgn_Stat_MCM/1  "pt_EngIgn_Stat_MCM"
  MCM21_MDEG_EURO_10ms_wrapper/65 -> pt_EngLoadIdx_Cval_PT/1  "pt_EngLoadIdx_Cval_PT"
  MCM21_MDEG_EURO_10ms_wrapper/66 -> pt_EngMode_Stat_MCM/1  "pt_EngMode_Stat_MCM"
  MCM21_MDEG_EURO_10ms_wrapper/67 -> pt_EngNO2RatioOut_Cval_MCM/1  "pt_EngNO2RatioOut_Cval_MCM"
  MCM21_MDEG_EURO_10ms_wrapper/68 -> pt_EngOilPress_Cval_MCM/1  "pt_EngOilPress_Cval_MCM"
  MCM21_MDEG_EURO_10ms_wrapper/69 -> pt_EngOpPnt_Stat_PT/1  "pt_EngOpPnt_Stat_PT"
  MCM21_MDEG_EURO_10ms_wrapper/70 -> pt_EngPendRls_Stat/1  "pt_EngPendRls_Stat"
  MCM21_MDEG_EURO_10ms_wrapper/71 -> pt_EngRegenRls_Stat/1  "pt_EngRegenRls_Stat"
  MCM21_MDEG_EURO_10ms_wrapper/72 -> pt_EngSpd_Cval_PT/1  "pt_EngSpd_Cval_PT"
  MCM21_MDEG_EURO_10ms_wrapper/73 -> pt_EngStSpInhbt_Rq_MCM/1  "pt_EngStSpInhbt_Rq_MCM"
  MCM21_MDEG_EURO_10ms_wrapper/74 -> pt_EngStrtr_Stat_MCM/1  "pt_EngStrtr_Stat_MCM"
  MCM21_MDEG_EURO_10ms_wrapper/75 -> pt_EngTransMd_Stat/1  "pt_EngTransMd_Stat"
  MCM21_MDEG_EURO_10ms_wrapper/76 -> pt_EngTrq_Cval_PT/1  "pt_EngTrq_Cval_PT"
  MCM21_MDEG_EURO_10ms_wrapper/77 -> pt_EngType_Cval_PT/1  "pt_EngType_Cval_PT"
  MCM21_MDEG_EURO_10ms_wrapper/78 -> pt_EngZeroTrq_Stat_MCM/1  "pt_EngZeroTrq_Stat_MCM"
  MCM21_MDEG_EURO_10ms_wrapper/79 -> pt_EomEng_Stat_MCM/1  "pt_EomEng_Stat_MCM"
  MCM21_MDEG_EURO_10ms_wrapper/80 -> pt_ExhGasMassFlowRate_Cval/1  "pt_ExhGasMassFlowRate_Cval"
  MCM21_MDEG_EURO_10ms_wrapper/81 -> pt_ExhGasOxyCont_Cval_PT/1  "pt_ExhGasOxyCont_Cval_PT"
  MCM21_MDEG_EURO_10ms_wrapper/82 -> pt_FuelMapSelNum_Cval_PT/1  "pt_FuelMapSelNum_Cval_PT"
  MCM21_MDEG_EURO_10ms_wrapper/83 -> pt_FuelMassFlowRate_Cval_PT/1  "pt_FuelMassFlowRate_Cval_PT"
  MCM21_MDEG_EURO_10ms_wrapper/84 -> pt_ISPRead30GNOxMd_MCM/1  "pt_ISPRead30GNOxMd_MCM"
  MCM21_MDEG_EURO_10ms_wrapper/85 -> pt_InertiaTrq_Cval_PT/1  "pt_InertiaTrq_Cval_PT"
  MCM21_MDEG_EURO_10ms_wrapper/86 -> pt_JakeBrk2_Stat_PT/1  "pt_JakeBrk2_Stat_PT"
  MCM21_MDEG_EURO_10ms_wrapper/87 -> pt_JakeBrk_Stat_PT/1  "pt_JakeBrk_Stat_PT"
  MCM21_MDEG_EURO_10ms_wrapper/88 -> pt_MCM_SglRes_Cval_PT/1  "pt_MCM_SglRes_Cval_PT"
  MCM21_MDEG_EURO_10ms_wrapper/89 -> pt_MaxActlEngTrq_Cval_PT/1  "pt_MaxActlEngTrq_Cval_PT"
  MCM21_MDEG_EURO_10ms_wrapper/90 -> pt_MaxActlRetTrq_Cval_PT/1  "pt_MaxActlRetTrq_Cval_PT"
  MCM21_MDEG_EURO_10ms_wrapper/91 -> pt_MaxEngBrkTrq_Cval_PT/1  "pt_MaxEngBrkTrq_Cval_PT"
  MCM21_MDEG_EURO_10ms_wrapper/92 -> pt_NOxMassFlowRate_Cval_PT/1  "pt_NOxMassFlowRate_Cval_PT"
  MCM21_MDEG_EURO_10ms_wrapper/93 -> pt_OilTemp_Cval_PT/1  "pt_OilTemp_Cval_PT"
  MCM21_MDEG_EURO_10ms_wrapper/94 -> pt_PM_MassFlowRate_Cval_PT/1  "pt_PM_MassFlowRate_Cval_PT"
  MCM21_MDEG_EURO_10ms_wrapper/95 -> pt_SmokeMdEOP_Stat/1  "pt_SmokeMdEOP_Stat"
  MCM21_MDEG_EURO_10ms_wrapper/96 -> pt_TankHt_Stat_PT/1  "pt_TankHt_Stat_PT"
  MCM21_MDEG_EURO_10ms_wrapper/97 -> pt_ThermoMgt_Stat_MCM/1  "pt_ThermoMgt_Stat_MCM"
  MCM21_MDEG_EURO_10ms_wrapper/98 -> pt_TrqLimNOx_Stat_PT/1  "pt_TrqLimNOx_Stat_PT"
  MCM21_MDEG_EURO_10ms_wrapper/99 -> pt_TrqLimPctAbsMax_Cval/1  "pt_TrqLimPctAbsMax_Cval"
  MCM21_MDEG_EURO_10ms_wrapper/100 -> pt_TrqLimPctCurve_Cval/1  "pt_TrqLimPctCurve_Cval"
  MCM21_MDEG_EURO_10ms_wrapper/101 -> pt_TurnOffDelayActBrk_Cval/1  "pt_TurnOffDelayActBrk_Cval"
  MCM21_MDEG_EURO_10ms_wrapper/102 -> pt_TurnOffDelayBrk1_Cval/1  "pt_TurnOffDelayBrk1_Cval"
  MCM21_MDEG_EURO_10ms_wrapper/103 -> pt_TurnOffDelayBrk2_Cval/1  "pt_TurnOffDelayBrk2_Cval"
  MCM21_MDEG_EURO_10ms_wrapper/104 -> pt_TurnOffDelayBrk3_Cval/1  "pt_TurnOffDelayBrk3_Cval"
  MCM21_MDEG_EURO_10ms_wrapper/105 -> pt_TurnOnDelayBrk1_Cval/1  "pt_TurnOnDelayBrk1_Cval"
  MCM21_MDEG_EURO_10ms_wrapper/106 -> pt_TurnOnDelayBrk2_Cval/1  "pt_TurnOnDelayBrk2_Cval"
  MCM21_MDEG_EURO_10ms_wrapper/107 -> pt_TurnOnDelayBrk3_Cval/1  "pt_TurnOnDelayBrk3_Cval"
  MCM21_MDEG_EURO_10ms_wrapper/108 -> pt_WFAMaxEngSpd30gNOx_MCM/1  "pt_WFAMaxEngSpd30gNOx_MCM"
  MCM21_MDEG_EURO_10ms_wrapper/109 -> pt_EngFrictTrq_Cval_PT/1  "pt_EngFrictTrq_Cval_PT"
  MCM21_MDEG_EURO_10ms_wrapper/110 -> pt_EngCylMd_Stat/1  "pt_EngCylMd_Stat"
  MCM21_MDEG_EURO_10ms_wrapper/111 -> mcm_brkflap_pos_des/1  "mcm_brkflap_pos_des"
  MCM21_MDEG_EURO_10ms_wrapper/112 -> pt_FuelMapNum_Cval_PT/1  "pt_FuelMapNum_Cval_PT"
  MCM21_MDEG_EURO_10ms_wrapper/113 -> pt_FuelMapEngSpd_Cval_PT/1  "pt_FuelMapEngSpd_Cval_PT"
  MCM21_MDEG_EURO_10ms_wrapper/114 -> pt_FuelMapTrq_Cval_PT/1  "pt_FuelMapTrq_Cval_PT"
  MCM21_MDEG_EURO_10ms_wrapper/115 -> pt_FuelMapTrqNoBst_Cval_PT/1  "pt_FuelMapTrqNoBst_Cval_PT"
  MCM21_MDEG_EURO_10ms_wrapper/116 -> mcm_act_braking_trq/1  "mcm_act_braking_trq"
  MCM21_MDEG_EURO_10ms_wrapper/117 -> mcm_trq_act_eff/1  "mcm_trq_act_eff"
  MCM21_MDEG_EURO_10ms_wrapper/118 -> mcm_fbf_des_fuel_mass/1  "mcm_fbf_des_fuel_mass"
  MCM21_MDEG_EURO_10ms_wrapper/119 -> mcm_tsa_itc_mode_act/1  "mcm_tsa_itc_mode_act"
  MCM21_MDEG_EURO_10ms_wrapper/120 -> mcm_wfa_wf_smoke/1  "mcm_wfa_wf_smoke"
  MCM21_MDEG_EURO_10ms_wrapper/121 -> mcm_fan_spd_req/1  "mcm_fan_spd_req"
  MCM21_MDEG_EURO_10ms_wrapper/122 -> mcm_starter_on/1  "mcm_starter_on"
  MCM21_MDEG_EURO_10ms_wrapper/123 -> pt_FuelCons_Cval_PT/1  "pt_FuelCons_Cval_PT"
  MCM21_MDEG_EURO_10ms_wrapper/124 -> pt_FanSpdPct_Cval_PT/1  "pt_FanSpdPct_Cval_PT"
  MCM21_MDEG_EURO_10ms_wrapper/125 -> pt_FanSpd_Cval_PT/1  "pt_FanSpd_Cval_PT"
  MCM21_MDEG_EURO_10ms_wrapper/126 -> mcm_am_sra3_current_position/1  "mcm_am_sra3_current_position"
  MCM21_MDEG_EURO_10ms_wrapper/127 -> mcm_am_sra3_des_pos/1  "mcm_am_sra3_des_pos"
  MCM21_MDEG_EURO_10ms_wrapper/128 -> mcm_ccf_act_air_mass/1  "mcm_ccf_act_air_mass"
  MCM21_MDEG_EURO_10ms_wrapper/129 -> mcm_EngNO2RatioOut_Cval_MCM/1  "mcm_EngNO2RatioOut_Cval_MCM"
  MCM21_MDEG_EURO_10ms_wrapper/130 -> mcm_NOxMassFlowRate_Cval_PT/1  "mcm_NOxMassFlowRate_Cval_PT"
  MCM21_MDEG_EURO_10ms_wrapper/131 -> mcm_EngFrictTrq_Cval_PT/1  "mcm_EngFrictTrq_Cval_PT"
  MCM21_MDEG_EURO_10ms_wrapper/132 -> pt_EngHours_Cval_PT/1  "pt_EngHours_Cval_PT"
  MCM21_MDEG_EURO_10ms_wrapper/133 -> mcm_EngSpd_Cval_PT/1  "mcm_EngSpd_Cval_PT"
  MCM21_MDEG_EURO_10ms_wrapper/134 -> mcm_EngTrq_Cval_PT/1  "mcm_EngTrq_Cval_PT"
  MCM21_MDEG_EURO_10ms_wrapper/135 -> pt_EngStrtrLk_Stat_MCM/1  "pt_EngStrtrLk_Stat_MCM"
  MCM21_MDEG_EURO_10ms_wrapper/136 -> pt_EngStrtrMode_Stat_MCM/1  "pt_EngStrtrMode_Stat_MCM"
  MCM21_MDEG_EURO_10ms_wrapper/137 -> pt_JBrakeSPointIdx_Cval/1  "pt_JBrakeSPointIdx_Cval"
  MCM21_MDEG_EURO_10ms_wrapper/138 -> pt_JBrakeSPointTrgtEngSpd_Cval/1  "pt_JBrakeSPointTrgtEngSpd_Cval"
  MCM21_MDEG_EURO_10ms_wrapper/139 -> pt_PwrClass_Cval_PT/1  "pt_PwrClass_Cval_PT"
  MCM21_MDEG_EURO_10ms_wrapper/140 -> pt_DeactDPF_ThermoMgt_Rq_PT/1  "pt_DeactDPF_ThermoMgt_Rq_PT"
  MCM21_MDEG_EURO_10ms_wrapper/141 -> pt_DelFMM_Rq_MCM/1  "pt_DelFMM_Rq_MCM"
  MCM21_MDEG_EURO_10ms_wrapper/142 -> pt_EngSNA_Stat_MCM/1  "pt_EngSNA_Stat_MCM"
  MCM21_MDEG_EURO_10ms_wrapper/143 -> pt_JBrakeSPointStrtEngSpd_Cval/1  "pt_JBrakeSPointStrtEngSpd_Cval"
  MCM21_MDEG_EURO_10ms_wrapper/144 -> pt_JBrakeWghtFac_Cval/1  "pt_JBrakeWghtFac_Cval"
  MCM21_MDEG_EURO_10ms_wrapper/145 -> pt_JBrkBPressStrtSpd1_3_Cval/1  "pt_JBrkBPressStrtSpd1_3_Cval"
  MCM21_MDEG_EURO_10ms_wrapper/146 -> pt_JBrkBPressStrtSpd1_6_Cval/1  "pt_JBrkBPressStrtSpd1_6_Cval"
  MCM21_MDEG_EURO_10ms_wrapper/147 -> pt_JBrkBPressStrtSpd2_3_Cval/1  "pt_JBrkBPressStrtSpd2_3_Cval"
  MCM21_MDEG_EURO_10ms_wrapper/148 -> pt_JBrkBPressStrtSpd2_6_Cval/1  "pt_JBrkBPressStrtSpd2_6_Cval"
  MCM21_MDEG_EURO_10ms_wrapper/149 -> pt_MC_C02_Cval_MCM/1  "pt_MC_C02_Cval_MCM"
  MCM21_MDEG_EURO_10ms_wrapper/150 -> pt_SysID_MCM/1  "pt_SysID_MCM"
  MCM21_MDEG_EURO_10ms_wrapper/151 -> mcm_intakethrottle_pos_des/1  "mcm_intakethrottle_pos_des"
  MCM21_MDEG_EURO_10ms_wrapper/152 -> pt_CoolTempIn_Cval_PT/1  "pt_CoolTempIn_Cval_PT"
  MCM21_MDEG_EURO_10ms_wrapper/153 -> pt_CoolTempOut_Cval_PT/1  "pt_CoolTempOut_Cval_PT"
  MCM21_MDEG_EURO_10ms_wrapper/154 -> mcm_mdot_SFI/1  "mcm_mdot_SFI"
  MCM21_MDEG_EURO_10ms_wrapper/155 -> pt_ChrgAirPressSens_Stat_PT/1  "pt_ChrgAirPressSens_Stat_PT"
  MCM21_MDEG_EURO_10ms_wrapper/156 -> pt_HC_DoserFlt_Stat/1  "pt_HC_DoserFlt_Stat"
  MCM21_MDEG_EURO_10ms_wrapper/157 -> pt_PM_MassFlowRate_Cval/1  "pt_PM_MassFlowRate_Cval"
  MCM21_MDEG_EURO_10ms_wrapper/158 -> pt_ExhHtSysRls_Stat/1  "pt_ExhHtSysRls_Stat"
  MCM21_MDEG_EURO_10ms_wrapper/159 -> pt_At1_IntkO2_Cval_MCM/1  "pt_At1_IntkO2_Cval_MCM"
  MCM21_MDEG_EURO_10ms_wrapper/160 -> pt_FuelDnstyCorrFctr_Cval/1  "pt_FuelDnstyCorrFctr_Cval"
  MCM21_MDEG_EURO_10ms_wrapper/161 -> pt_TurboOutTemp_Cval/1  "pt_TurboOutTemp_Cval"
  MCM21_MDEG_EURO_10ms_wrapper/162 -> pt_ExhGasFlwRateMod_Cval_MCM/1  "pt_ExhGasFlwRateMod_Cval_MCM"
  MCM21_MDEG_EURO_10ms_wrapper/163 -> pt_BaroPress_Cval_MCM/1  "pt_BaroPress_Cval_MCM"
  MCM21_MDEG_EURO_10ms_wrapper/164 -> pt_Tier4Induce_Stat/1  "pt_Tier4Induce_Stat"
  MCM21_MDEG_EURO_10ms_wrapper/165 -> pt_Tier4Induce_FR_Cval_MCM/1  "pt_Tier4Induce_FR_Cval_MCM"
  MCM21_MDEG_EURO_10ms_wrapper/166 -> pt_Tier4InduceOvrd_Stat/1  "pt_Tier4InduceOvrd_Stat"
  MCM21_MDEG_EURO_10ms_wrapper/167 -> pt_CfgBit2_Cval_MCM/1  "pt_CfgBit2_Cval_MCM"
  MCM21_MDEG_EURO_10ms_wrapper/168 -> pt_CfgBit_Cval_MCM/1  "pt_CfgBit_Cval_MCM"
  MCM21_MDEG_EURO_10ms_wrapper/169 -> pt_MCM_SglRes2_Cval_PT/1  "pt_MCM_SglRes2_Cval_PT"
  MCM21_MDEG_EURO_10ms_wrapper/170 -> pt_WtrInjQuant_Cval/1  "pt_WtrInjQuant_Cval"
  MCM21_MDEG_EURO_10ms_wrapper/171 -> pt_CfgBit2_extd_Cval_MCM/1  "pt_CfgBit2_extd_Cval_MCM"
  MCM21_MDEG_EURO_10ms_wrapper/172 -> pt_DEF_Lmp_Stat_PT/1  "pt_DEF_Lmp_Stat_PT"
  MCM21_MDEG_EURO_10ms_wrapper/173 -> mcm_EomEng_Stat_MCM/1  "mcm_EomEng_Stat_MCM"
  MCM21_MDEG_EURO_10ms_wrapper/174 -> pt_EngCoolTemp_Cval_MCM/1  "pt_EngCoolTemp_Cval_MCM"
  MCM21_MDEG_EURO_10ms_wrapper/175 -> mcm_eaf_nox_content_cor/1  "mcm_eaf_nox_content_cor"
  MCM21_MDEG_EURO_10ms_wrapper/176 -> pt_ThermoRoll_Rq/1  "pt_ThermoRoll_Rq"
  MCM21_MDEG_EURO_10ms_wrapper/177 -> mcm_am_sra4_des_pos/1  "mcm_am_sra4_des_pos"
  MCM21_MDEG_EURO_10ms_wrapper/178 -> mcm_pwm_wp/1  "mcm_pwm_wp"
